simulink model "w2_warplab_trigger_proc"  (Simulink 7.7)
settings: Solver=ode45  StartTime=0.0  StopTime=1000  RelTol=1e-3
InitFcn:
  | w2_warplab_trigger_proc_init
StartFcn:
  | w2_warplab_trigger_proc_init
undefined symbols (not defined in the file or in its folder): gcbh, xlBlockLoadCallback, xlGetNormalizedPeriod
libraries: xbsIndex_r4 x819, simulink x1
(part 3 of 6)

== system w2_warplab_trigger_proc/Pulse Extender (4 cycles) ==
  IN : Inport
  Logical : xbsIndex_r4/Logical  logical_function=OR  inputs=4  en=off  latency=0  precision=Full  arith_type=Unsigned  n_bits=16  bin_pt=0  align_bp=on  dbl_ovrd=off  block_type=logical
      settings: xl_area=[1 0 0 1 0 0 0]  block_version=VER_STRING_GOES_HERE
  Register1 : xbsIndex_r4/Register  init=0  rst=off  en=off  dbl_ovrd=off  block_type=register
  Register2 : xbsIndex_r4/Register  init=0  rst=off  en=off  dbl_ovrd=off  block_type=register
  Register3 : xbsIndex_r4/Register  init=0  rst=off  en=off  dbl_ovrd=off  block_type=register
  OUT : Outport
  wires:
  Logical/1 -> OUT/1
  IN/1 -> Logical/1, Register1/1
  Register1/1 -> Logical/2, Register2/1
  Register2/1 -> Logical/3, Register3/1
  Register3/1 -> Logical/4

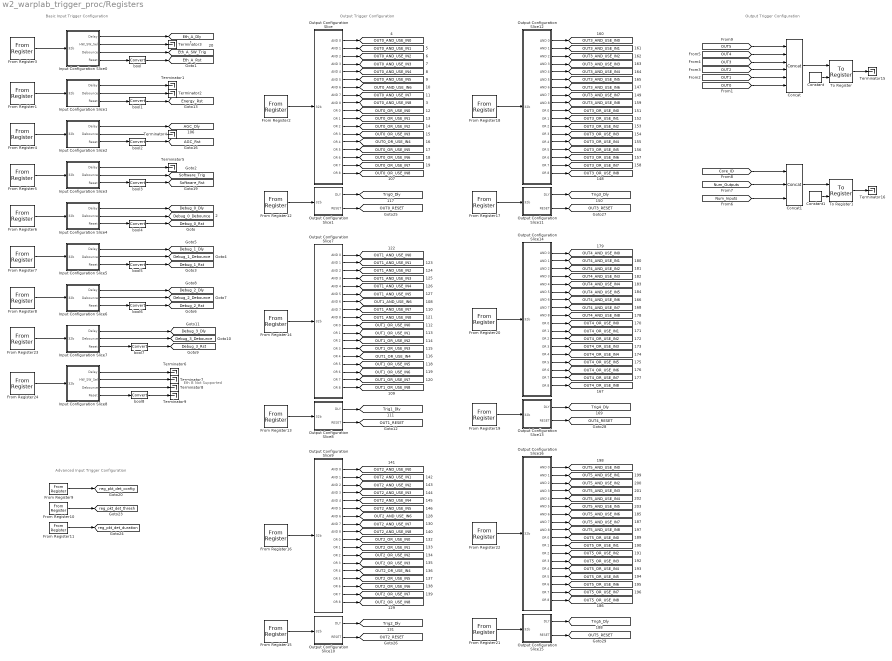
== system w2_warplab_trigger_proc/Registers ==
  note: Basic Input Trigger Configuration
  note: Advanced Input Trigger Configuration
  note: Output Trigger Configuration
  note: Output Trigger Configuration
  note: Eth B Not Supported
  Concat : xbsIndex_r4/Concat  num_inputs=6  dbl_ovrd=off  block_type=concat
  Concat1 : xbsIndex_r4/Concat  num_inputs=3  dbl_ovrd=off  block_type=concat
  Constant : xbsIndex_r4/Constant  const=1  gui_display_data_type=Boolean  arith_type=Boolean  n_bits=16  bin_pt=14  preci_type=Single  exp_width=8  frac_width=24  explicit_period=off  period=1  equ=P=C  opselect=C  inp2=PCIN>>17  opr=+  inp1=P  carry=CIN  dbl_ovrd=off  block_type=constant
  Constant1 : xbsIndex_r4/Constant  const=1  gui_display_data_type=Boolean  arith_type=Boolean  n_bits=16  bin_pt=14  preci_type=Single  exp_width=8  frac_width=24  explicit_period=off  period=1  equ=P=C  opselect=C  inp2=PCIN>>17  opr=+  inp1=P  carry=CIN  dbl_ovrd=off  block_type=constant
  From Register1 : xbsIndex_r4/From Register  shared_memory_name='TRIG_IN_CONF_1'  init=TRIG_IN_CONF_1  period=1  ownership=Locally owned and initialized  gui_display_data_type=Fixed-point  arith_type=Unsigned  n_bits=32  bin_pt=0  preci_type=Single  dbl_ovrd=off  block_type=fromreg
      settings: AttributesFormatString=<< %<shared_memory_name> >>  infoedit="Register block that reads data to a shared memory register.  Delay of one sample period."
  From Register10 : xbsIndex_r4/From Register  shared_memory_name='RSSI_PKT_DET_THRESHOLDS'  init=RSSI_PKT_DET_THRESHOLDS  period=1  ownership=Locally owned and initialized  gui_display_data_type=Fixed-point  arith_type=Unsigned  n_bits=32  bin_pt=0  preci_type=Single  dbl_ovrd=off  block_type=fromreg
      settings: AttributesFormatString=<< %<shared_memory_name> >>  infoedit="Register block that reads data to a shared memory register.  Delay of one sample period."  block_version=8.2
  From Register11 : xbsIndex_r4/From Register  shared_memory_name='RSSI_PKT_DET_DURATIONS'  init=RSSI_PKT_DET_DURATIONS  period=1  ownership=Locally owned and initialized  gui_display_data_type=Fixed-point  arith_type=Unsigned  n_bits=32  bin_pt=0  preci_type=Single  dbl_ovrd=off  block_type=fromreg
      settings: AttributesFormatString=<< %<shared_memory_name> >>  infoedit="Register block that reads data to a shared memory register.  Delay of one sample period."  block_version=8.2
  From Register12 : xbsIndex_r4/From Register  shared_memory_name='TRIG_OUT_0_CONF_1'  init=TRIG_OUT_0_CONF_1  period=1  ownership=Locally owned and initialized  gui_display_data_type=Fixed-point  arith_type=Unsigned  n_bits=32  bin_pt=0  preci_type=Single  dbl_ovrd=off  block_type=fromreg
      settings: AttributesFormatString=<< %<shared_memory_name> >>  infoedit="Register block that reads data to a shared memory register.  Delay of one sample period."
  From Register13 : xbsIndex_r4/From Register  shared_memory_name='TRIG_OUT_1_CONF_1'  init=TRIG_OUT_1_CONF_1  period=1  ownership=Locally owned and initialized  gui_display_data_type=Fixed-point  arith_type=Unsigned  n_bits=32  bin_pt=0  preci_type=Single  dbl_ovrd=off  block_type=fromreg
      settings: AttributesFormatString=<< %<shared_memory_name> >>  infoedit="Register block that reads data to a shared memory register.  Delay of one sample period."
  From Register14 : xbsIndex_r4/From Register  shared_memory_name='TRIG_OUT_1_CONF_0'  init=TRIG_OUT_1_CONF_0  period=1  ownership=Locally owned and initialized  gui_display_data_type=Fixed-point  arith_type=Unsigned  n_bits=32  bin_pt=0  preci_type=Single  dbl_ovrd=off  block_type=fromreg
      settings: AttributesFormatString=<< %<shared_memory_name> >>  infoedit="Register block that reads data to a shared memory register.  Delay of one sample period."
  From Register15 : xbsIndex_r4/From Register  shared_memory_name='TRIG_OUT_2_CONF_1'  init=TRIG_OUT_2_CONF_1  period=1  ownership=Locally owned and initialized  gui_display_data_type=Fixed-point  arith_type=Unsigned  n_bits=32  bin_pt=0  preci_type=Single  dbl_ovrd=off  block_type=fromreg
      settings: AttributesFormatString=<< %<shared_memory_name> >>  infoedit="Register block that reads data to a shared memory register.  Delay of one sample period."
  From Register16 : xbsIndex_r4/From Register  shared_memory_name='TRIG_OUT_2_CONF_0'  init=TRIG_OUT_2_CONF_0  period=1  ownership=Locally owned and initialized  gui_display_data_type=Fixed-point  arith_type=Unsigned  n_bits=32  bin_pt=0  preci_type=Single  dbl_ovrd=off  block_type=fromreg
      settings: AttributesFormatString=<< %<shared_memory_name> >>  infoedit="Register block that reads data to a shared memory register.  Delay of one sample period."
  From Register17 : xbsIndex_r4/From Register  shared_memory_name='TRIG_OUT_3_CONF_1'  init=TRIG_OUT_3_CONF_1  period=1  ownership=Locally owned and initialized  gui_display_data_type=Fixed-point  arith_type=Unsigned  n_bits=32  bin_pt=0  preci_type=Single  dbl_ovrd=off  block_type=fromreg
      settings: AttributesFormatString=<< %<shared_memory_name> >>  infoedit="Register block that reads data to a shared memory register.  Delay of one sample period."
  From Register18 : xbsIndex_r4/From Register  shared_memory_name='TRIG_OUT_3_CONF_0'  init=TRIG_OUT_3_CONF_0  period=1  ownership=Locally owned and initialized  gui_display_data_type=Fixed-point  arith_type=Unsigned  n_bits=32  bin_pt=0  preci_type=Single  dbl_ovrd=off  block_type=fromreg
      settings: AttributesFormatString=<< %<shared_memory_name> >>  infoedit="Register block that reads data to a shared memory register.  Delay of one sample period."
  From Register19 : xbsIndex_r4/From Register  shared_memory_name='TRIG_OUT_4_CONF_1'  init=TRIG_OUT_4_CONF_1  period=1  ownership=Locally owned and initialized  gui_display_data_type=Fixed-point  arith_type=Unsigned  n_bits=32  bin_pt=0  preci_type=Single  dbl_ovrd=off  block_type=fromreg
      settings: AttributesFormatString=<< %<shared_memory_name> >>  infoedit="Register block that reads data to a shared memory register.  Delay of one sample period."
  From Register2 : xbsIndex_r4/From Register  shared_memory_name='TRIG_OUT_0_CONF_0'  init=TRIG_OUT_0_CONF_0  period=1  ownership=Locally owned and initialized  gui_display_data_type=Fixed-point  arith_type=Unsigned  n_bits=32  bin_pt=0  preci_type=Single  dbl_ovrd=off  block_type=fromreg
      settings: AttributesFormatString=<< %<shared_memory_name> >>  infoedit="Register block that reads data to a shared memory register.  Delay of one sample period."
  From Register20 : xbsIndex_r4/From Register  shared_memory_name='TRIG_OUT_4_CONF_0'  init=TRIG_OUT_4_CONF_0  period=1  ownership=Locally owned and initialized  gui_display_data_type=Fixed-point  arith_type=Unsigned  n_bits=32  bin_pt=0  preci_type=Single  dbl_ovrd=off  block_type=fromreg
      settings: AttributesFormatString=<< %<shared_memory_name> >>  infoedit="Register block that reads data to a shared memory register.  Delay of one sample period."
  From Register21 : xbsIndex_r4/From Register  shared_memory_name='TRIG_OUT_5_CONF_1'  init=TRIG_OUT_5_CONF_1  period=1  ownership=Locally owned and initialized  gui_display_data_type=Fixed-point  arith_type=Unsigned  n_bits=32  bin_pt=0  preci_type=Single  dbl_ovrd=off  block_type=fromreg
      settings: AttributesFormatString=<< %<shared_memory_name> >>  infoedit="Register block that reads data to a shared memory register.  Delay of one sample period."
  From Register22 : xbsIndex_r4/From Register  shared_memory_name='TRIG_OUT_5_CONF_0'  init=TRIG_OUT_5_CONF_0  period=1  ownership=Locally owned and initialized  gui_display_data_type=Fixed-point  arith_type=Unsigned  n_bits=32  bin_pt=0  preci_type=Single  dbl_ovrd=off  block_type=fromreg
      settings: AttributesFormatString=<< %<shared_memory_name> >>  infoedit="Register block that reads data to a shared memory register.  Delay of one sample period."
  From Register23 : xbsIndex_r4/From Register  shared_memory_name='TRIG_IN_CONF_7'  init=TRIG_IN_CONF_7  period=1  ownership=Locally owned and initialized  gui_display_data_type=Fixed-point  arith_type=Unsigned  n_bits=32  bin_pt=0  preci_type=Single  dbl_ovrd=off  block_type=fromreg
      settings: AttributesFormatString=<< %<shared_memory_name> >>  infoedit="Register block that reads data to a shared memory register.  Delay of one sample period."
  From Register24 : xbsIndex_r4/From Register  shared_memory_name='TRIG_IN_CONF_8'  init=TRIG_IN_CONF_8  period=1  ownership=Locally owned and initialized  gui_display_data_type=Fixed-point  arith_type=Unsigned  n_bits=32  bin_pt=0  preci_type=Single  dbl_ovrd=off  block_type=fromreg
      settings: AttributesFormatString=<< %<shared_memory_name> >>  infoedit="Register block that reads data to a shared memory register.  Delay of one sample period."
  From Register3 : xbsIndex_r4/From Register  shared_memory_name='TRIG_IN_CONF_0'  init=TRIG_IN_CONF_0  period=1  ownership=Locally owned and initialized  gui_display_data_type=Fixed-point  arith_type=Unsigned  n_bits=32  bin_pt=0  preci_type=Single  dbl_ovrd=off  block_type=fromreg
      settings: AttributesFormatString=<< %<shared_memory_name> >>  infoedit="Register block that reads data to a shared memory register.  Delay of one sample period."
  From Register4 : xbsIndex_r4/From Register  shared_memory_name='TRIG_IN_CONF_2'  init=TRIG_IN_CONF_2  period=1  ownership=Locally owned and initialized  gui_display_data_type=Fixed-point  arith_type=Unsigned  n_bits=32  bin_pt=0  preci_type=Single  dbl_ovrd=off  block_type=fromreg
      settings: AttributesFormatString=<< %<shared_memory_name> >>  infoedit="Register block that reads data to a shared memory register.  Delay of one sample period."
  From Register5 : xbsIndex_r4/From Register  shared_memory_name='TRIG_IN_CONF_3'  init=TRIG_IN_CONF_3  period=1  ownership=Locally owned and initialized  gui_display_data_type=Fixed-point  arith_type=Unsigned  n_bits=32  bin_pt=0  preci_type=Single  dbl_ovrd=off  block_type=fromreg
      settings: AttributesFormatString=<< %<shared_memory_name> >>  infoedit="Register block that reads data to a shared memory register.  Delay of one sample period."
  From Register6 : xbsIndex_r4/From Register  shared_memory_name='TRIG_IN_CONF_4'  init=TRIG_IN_CONF_4  period=1  ownership=Locally owned and initialized  gui_display_data_type=Fixed-point  arith_type=Unsigned  n_bits=32  bin_pt=0  preci_type=Single  dbl_ovrd=off  block_type=fromreg
      settings: AttributesFormatString=<< %<shared_memory_name> >>  infoedit="Register block that reads data to a shared memory register.  Delay of one sample period."
  From Register7 : xbsIndex_r4/From Register  shared_memory_name='TRIG_IN_CONF_5'  init=TRIG_IN_CONF_5  period=1  ownership=Locally owned and initialized  gui_display_data_type=Fixed-point  arith_type=Unsigned  n_bits=32  bin_pt=0  preci_type=Single  dbl_ovrd=off  block_type=fromreg
      settings: AttributesFormatString=<< %<shared_memory_name> >>  infoedit="Register block that reads data to a shared memory register.  Delay of one sample period."
  From Register8 : xbsIndex_r4/From Register  shared_memory_name='TRIG_IN_CONF_6'  init=TRIG_IN_CONF_6  period=1  ownership=Locally owned and initialized  gui_display_data_type=Fixed-point  arith_type=Unsigned  n_bits=32  bin_pt=0  preci_type=Single  dbl_ovrd=off  block_type=fromreg
      settings: AttributesFormatString=<< %<shared_memory_name> >>  infoedit="Register block that reads data to a shared memory register.  Delay of one sample period."
  From Register9 : xbsIndex_r4/From Register  shared_memory_name='RSSI_PKT_DET_CONFIG'  init=RSSI_PKT_DET_CONFIG  period=1  ownership=Locally owned and initialized  gui_display_data_type=Fixed-point  arith_type=Unsigned  n_bits=32  bin_pt=0  preci_type=Single  dbl_ovrd=off  block_type=fromreg
      settings: AttributesFormatString=<< %<shared_memory_name> >>  infoedit="Register block that reads data to a shared memory register.  Delay of one sample period."  block_version=8.2
  Input Configuration Slice0 : Subsystem
  Input Configuration Slice1 : Subsystem
  Input Configuration Slice2 : Subsystem
  Input Configuration Slice3 : Subsystem
  Input Configuration Slice4 : Subsystem
  Input Configuration Slice5 : Subsystem
  Input Configuration Slice6 : Subsystem
  Input Configuration Slice7 : Subsystem
  Input Configuration Slice8 : Subsystem
  Output Configuration Slice : Subsystem
  Output Configuration Slice1 : Subsystem
  Output Configuration Slice10 : Subsystem
  Output Configuration Slice11 : Subsystem
  Output Configuration Slice12 : Subsystem
  Output Configuration Slice13 : Subsystem
  Output Configuration Slice14 : Subsystem
  Output Configuration Slice15 : Subsystem
  Output Configuration Slice16 : Subsystem
  Output Configuration Slice7 : Subsystem
  Output Configuration Slice8 : Subsystem
  Output Configuration Slice9 : Subsystem
  Terminator{1..9,15..16} (11 alike) : Terminator
  To Register : xbsIndex_r4/To Register  shared_memory_name='TRIG_OUT'  init=0  ownership=Locally owned and initialized  explicit_data_type=on  gui_display_data_type=Fixed-point  arith_type=Unsigned  n_bits=6  bin_pt=0  preci_type=Single  dbl_ovrd=off  block_type=toreg
      settings: AttributesFormatString=<< %<shared_memory_name> >>  infoedit="Register block that writes data to a shared memory register.  Delay of one sample period."
  To Register1 : xbsIndex_r4/To Register  shared_memory_name='CORE_INFO'  init=0  ownership=Locally owned and initialized  explicit_data_type=on  gui_display_data_type=Fixed-point  arith_type=Unsigned  n_bits=24  bin_pt=0  preci_type=Single  dbl_ovrd=off  block_type=toreg
      settings: AttributesFormatString=<< %<shared_memory_name> >>  infoedit="Register block that writes data to a shared memory register.  Delay of one sample period."
  bool{,1..8} (9 alike) : xbsIndex_r4/Convert  gui_display_data_type=Boolean  arith_type=Boolean  n_bits=16  bin_pt=14  float_type=Single  exp_bits=8  fraction_bits=24  quantization=Truncate  overflow=Wrap  en=off  latency=0  dbl_ovrd=off  pipeline=off  block_type=convert
  tag scope: AGC_Dly=global, AGC_Rst=global, Debug_0_Debounce=global, Debug_0_Dly=global, Debug_0_Rst=global, Debug_1_Debounce=global, Debug_1_Dly=global, Debug_1_Rst=global, Debug_2_Debounce=global, Debug_2_Dly=global, Debug_2_Rst=global, Debug_3_Debounce=global, Debug_3_Dly=global, Debug_3_Rst=global, Energy_Rst=global, Eth_A_Dly=global, Eth_A_Rst=global, Eth_A_SW_Trig=global, OUT0_AND_USE_IN0=global, OUT0_AND_USE_IN1=global, OUT0_AND_USE_IN2=global, OUT0_AND_USE_IN3=global, OUT0_AND_USE_IN4=global, OUT0_AND_USE_IN5=global, OUT0_AND_USE_IN6=global, OUT0_AND_USE_IN7=global, OUT0_AND_USE_IN8=global, OUT0_OR_USE_IN0=global, OUT0_OR_USE_IN1=global, OUT0_OR_USE_IN2=global, OUT0_OR_USE_IN3=global, OUT0_OR_USE_IN4=global, OUT0_OR_USE_IN5=global, OUT0_OR_USE_IN6=global, OUT0_OR_USE_IN7=global, OUT0_OR_USE_IN8=global, OUT0_RESET=global, OUT1_AND_USE_IN0=global, OUT1_AND_USE_IN1=global, OUT1_AND_USE_IN2=global, OUT1_AND_USE_IN3=global, OUT1_AND_USE_IN4=global, OUT1_AND_USE_IN5=global, OUT1_AND_USE_IN6=global, OUT1_AND_USE_IN7=global, OUT1_AND_USE_IN8=global, OUT1_OR_USE_IN0=global, OUT1_OR_USE_IN1=global, OUT1_OR_USE_IN2=global, OUT1_OR_USE_IN3=global, OUT1_OR_USE_IN4=global, OUT1_OR_USE_IN5=global, OUT1_OR_USE_IN6=global, OUT1_OR_USE_IN7=global, OUT1_OR_USE_IN8=global, OUT1_RESET=global, OUT2_AND_USE_IN0=global, OUT2_AND_USE_IN1=global, OUT2_AND_USE_IN2=global, OUT2_AND_USE_IN3=global, OUT2_AND_USE_IN4=global, OUT2_AND_USE_IN5=global, OUT2_AND_USE_IN6=global, OUT2_AND_USE_IN7=global, OUT2_AND_USE_IN8=global, OUT2_OR_USE_IN0=global, OUT2_OR_USE_IN1=global, OUT2_OR_USE_IN2=global, OUT2_OR_USE_IN3=global, OUT2_OR_USE_IN4=global, OUT2_OR_USE_IN5=global, OUT2_OR_USE_IN6=global, OUT2_OR_USE_IN7=global, OUT2_OR_USE_IN8=global, OUT2_RESET=global, OUT3_AND_USE_IN0=global, OUT3_AND_USE_IN1=global, OUT3_AND_USE_IN2=global, OUT3_AND_USE_IN3=global, OUT3_AND_USE_IN4=global, OUT3_AND_USE_IN5=global, OUT3_AND_USE_IN6=global, OUT3_AND_USE_IN7=global, OUT3_AND_USE_IN8=global, OUT3_OR_USE_IN0=global, OUT3_OR_USE_IN1=global, OUT3_OR_USE_IN2=global, OUT3_OR_USE_IN3=global, OUT3_OR_USE_IN4=global, OUT3_OR_USE_IN5=global, OUT3_OR_USE_IN6=global, OUT3_OR_USE_IN7=global, OUT3_OR_USE_IN8=global, OUT3_RESET=global, OUT4_AND_USE_IN0=global, OUT4_AND_USE_IN1=global, OUT4_AND_USE_IN2=global, OUT4_AND_USE_IN3=global, OUT4_AND_USE_IN4=global, OUT4_AND_USE_IN5=global, OUT4_AND_USE_IN6=global, OUT4_AND_USE_IN7=global, OUT4_AND_USE_IN8=global, OUT4_OR_USE_IN0=global, OUT4_OR_USE_IN1=global, OUT4_OR_USE_IN2=global, OUT4_OR_USE_IN3=global, OUT4_OR_USE_IN4=global, OUT4_OR_USE_IN5=global, OUT4_OR_USE_IN6=global, OUT4_OR_USE_IN7=global, OUT4_OR_USE_IN8=global, OUT4_RESET=global, OUT5_AND_USE_IN0=global, OUT5_AND_USE_IN1=global, OUT5_AND_USE_IN2=global, OUT5_AND_USE_IN3=global, OUT5_AND_USE_IN4=global, OUT5_AND_USE_IN5=global, OUT5_AND_USE_IN6=global, OUT5_AND_USE_IN7=global, OUT5_AND_USE_IN8=global, OUT5_OR_USE_IN0=global, OUT5_OR_USE_IN1=global, OUT5_OR_USE_IN2=global, OUT5_OR_USE_IN3=global, OUT5_OR_USE_IN4=global, OUT5_OR_USE_IN5=global, OUT5_OR_USE_IN6=global, OUT5_OR_USE_IN7=global, OUT5_OR_USE_IN8=global, OUT5_RESET=global, Software_Rst=global, Software_Trig=global, Trig0_Dly=global, Trig1_Dly=global, Trig2_Dly=global, Trig3_Dly=global, Trig4_Dly=global, Trig5_Dly=global, reg_pkt_det_config=global, reg_pkt_det_duration=global, reg_pkt_det_thresh=global
  wires:
  From Register9/1 -> [reg_pkt_det_config]
  From Register10/1 -> [reg_pkt_det_thresh]
  From Register11/1 -> [reg_pkt_det_duration]
  From Register2/1 -> Output Configuration Slice/1(32b)
  Output Configuration Slice/1(AND 0) -> [OUT0_AND_USE_IN0]
  Output Configuration Slice/2(AND 1) -> [OUT0_AND_USE_IN1]
  Output Configuration Slice/3(AND 2) -> [OUT0_AND_USE_IN2]
  Output Configuration Slice/4(AND 3) -> [OUT0_AND_USE_IN3]
  Output Configuration Slice/5(AND 4) -> [OUT0_AND_USE_IN4]
  Output Configuration Slice/6(AND 5) -> [OUT0_AND_USE_IN5]
  Output Configuration Slice/7(AND 6) -> [OUT0_AND_USE_IN6]
  Output Configuration Slice/8(AND 7) -> [OUT0_AND_USE_IN7]
  Output Configuration Slice/10(OR 0) -> [OUT0_OR_USE_IN0]
  Output Configuration Slice/11(OR 1) -> [OUT0_OR_USE_IN1]
  Output Configuration Slice/12(OR 2) -> [OUT0_OR_USE_IN2]
  Output Configuration Slice/13(OR 3) -> [OUT0_OR_USE_IN3]
  Output Configuration Slice/14(OR 4) -> [OUT0_OR_USE_IN4]
  Output Configuration Slice/15(OR 5) -> [OUT0_OR_USE_IN5]
  Output Configuration Slice/16(OR 6) -> [OUT0_OR_USE_IN6]
  Output Configuration Slice/17(OR 7) -> [OUT0_OR_USE_IN7]
  [OUT4] -> Concat/2
  [OUT3] -> Concat/3
  [OUT2] -> Concat/4
  [OUT1] -> Concat/5
  [OUT0] -> Concat/6
  Concat/1 -> To Register/1
  Constant/1 -> To Register/2
  Concat1/1 -> To Register1/1
  Constant1/1 -> To Register1/2
  [Core_ID] -> Concat1/1
  [Num_Outputs] -> Concat1/2
  [Num_Inputs] -> Concat1/3
  Output Configuration Slice/9(AND 8) -> [OUT0_AND_USE_IN8]
  Output Configuration Slice/18(OR 8) -> [OUT0_OR_USE_IN8]
  From Register14/1 -> Output Configuration Slice7/1(32b)
  Output Configuration Slice7/1(AND 0) -> [OUT1_AND_USE_IN0]
  Output Configuration Slice7/2(AND 1) -> [OUT1_AND_USE_IN1]
  Output Configuration Slice7/3(AND 2) -> [OUT1_AND_USE_IN2]
  Output Configuration Slice7/4(AND 3) -> [OUT1_AND_USE_IN3]
  Output Configuration Slice7/5(AND 4) -> [OUT1_AND_USE_IN4]
  Output Configuration Slice7/6(AND 5) -> [OUT1_AND_USE_IN5]
  Output Configuration Slice7/7(AND 6) -> [OUT1_AND_USE_IN6]
  Output Configuration Slice7/8(AND 7) -> [OUT1_AND_USE_IN7]
  Output Configuration Slice7/10(OR 0) -> [OUT1_OR_USE_IN0]
  Output Configuration Slice7/11(OR 1) -> [OUT1_OR_USE_IN1]
  Output Configuration Slice7/12(OR 2) -> [OUT1_OR_USE_IN2]
  Output Configuration Slice7/13(OR 3) -> [OUT1_OR_USE_IN3]
  Output Configuration Slice7/14(OR 4) -> [OUT1_OR_USE_IN4]
  Output Configuration Slice7/15(OR 5) -> [OUT1_OR_USE_IN5]
  Output Configuration Slice7/16(OR 6) -> [OUT1_OR_USE_IN6]
  Output Configuration Slice7/17(OR 7) -> [OUT1_OR_USE_IN7]
  From Register13/1 -> Output Configuration Slice8/1(32b)
  Output Configuration Slice8/2(RESET) -> [OUT1_RESET]
  Output Configuration Slice8/1(DLY) -> [Trig1_Dly]
  Output Configuration Slice7/9(AND 8) -> [OUT1_AND_USE_IN8]
  Output Configuration Slice7/18(OR 8) -> [OUT1_OR_USE_IN8]
  From Register16/1 -> Output Configuration Slice9/1(32b)
  Output Configuration Slice9/1(AND 0) -> [OUT2_AND_USE_IN0]
  Output Configuration Slice9/2(AND 1) -> [OUT2_AND_USE_IN1]
  Output Configuration Slice9/3(AND 2) -> [OUT2_AND_USE_IN2]
  Output Configuration Slice9/4(AND 3) -> [OUT2_AND_USE_IN3]
  Output Configuration Slice9/5(AND 4) -> [OUT2_AND_USE_IN4]
  Output Configuration Slice9/6(AND 5) -> [OUT2_AND_USE_IN5]
  Output Configuration Slice9/7(AND 6) -> [OUT2_AND_USE_IN6]
  Output Configuration Slice9/8(AND 7) -> [OUT2_AND_USE_IN7]
  Output Configuration Slice9/10(OR 0) -> [OUT2_OR_USE_IN0]
  Output Configuration Slice9/11(OR 1) -> [OUT2_OR_USE_IN1]
  Output Configuration Slice9/12(OR 2) -> [OUT2_OR_USE_IN2]
  Output Configuration Slice9/13(OR 3) -> [OUT2_OR_USE_IN3]
  Output Configuration Slice9/14(OR 4) -> [OUT2_OR_USE_IN4]
  Output Configuration Slice9/15(OR 5) -> [OUT2_OR_USE_IN5]
  Output Configuration Slice9/16(OR 6) -> [OUT2_OR_USE_IN6]
  Output Configuration Slice9/17(OR 7) -> [OUT2_OR_USE_IN7]
  From Register15/1 -> Output Configuration Slice10/1(32b)
  Output Configuration Slice10/2(RESET) -> [OUT2_RESET]
  Output Configuration Slice10/1(DLY) -> [Trig2_Dly]
  Output Configuration Slice9/9(AND 8) -> [OUT2_AND_USE_IN8]
  Output Configuration Slice9/18(OR 8) -> [OUT2_OR_USE_IN8]
  From Register18/1 -> Output Configuration Slice12/1(32b)
  Output Configuration Slice12/1(AND 0) -> [OUT3_AND_USE_IN0]
  Output Configuration Slice12/2(AND 1) -> [OUT3_AND_USE_IN1]
  Output Configuration Slice12/3(AND 2) -> [OUT3_AND_USE_IN2]
  Output Configuration Slice12/4(AND 3) -> [OUT3_AND_USE_IN3]
  Output Configuration Slice12/5(AND 4) -> [OUT3_AND_USE_IN4]
  Output Configuration Slice12/6(AND 5) -> [OUT3_AND_USE_IN5]
  Output Configuration Slice12/7(AND 6) -> [OUT3_AND_USE_IN6]
  Output Configuration Slice12/8(AND 7) -> [OUT3_AND_USE_IN7]
  Output Configuration Slice12/10(OR 0) -> [OUT3_OR_USE_IN0]
  Output Configuration Slice12/11(OR 1) -> [OUT3_OR_USE_IN1]
  Output Configuration Slice12/12(OR 2) -> [OUT3_OR_USE_IN2]
  Output Configuration Slice12/13(OR 3) -> [OUT3_OR_USE_IN3]
  Output Configuration Slice12/14(OR 4) -> [OUT3_OR_USE_IN4]
  Output Configuration Slice12/15(OR 5) -> [OUT3_OR_USE_IN5]
  Output Configuration Slice12/16(OR 6) -> [OUT3_OR_USE_IN6]
  Output Configuration Slice12/17(OR 7) -> [OUT3_OR_USE_IN7]
  From Register17/1 -> Output Configuration Slice11/1(32b)
  Output Configuration Slice11/2(RESET) -> [OUT3_RESET]
  Output Configuration Slice11/1(DLY) -> [Trig3_Dly]
  Output Configuration Slice12/9(AND 8) -> [OUT3_AND_USE_IN8]
  Output Configuration Slice12/18(OR 8) -> [OUT3_OR_USE_IN8]
  From Register20/1 -> Output Configuration Slice14/1(32b)
  Output Configuration Slice14/1(AND 0) -> [OUT4_AND_USE_IN0]
  Output Configuration Slice14/2(AND 1) -> [OUT4_AND_USE_IN1]
  Output Configuration Slice14/3(AND 2) -> [OUT4_AND_USE_IN2]
  Output Configuration Slice14/4(AND 3) -> [OUT4_AND_USE_IN3]
  Output Configuration Slice14/5(AND 4) -> [OUT4_AND_USE_IN4]
  Output Configuration Slice14/6(AND 5) -> [OUT4_AND_USE_IN5]
  Output Configuration Slice14/7(AND 6) -> [OUT4_AND_USE_IN6]
  Output Configuration Slice14/8(AND 7) -> [OUT4_AND_USE_IN7]
  Output Configuration Slice14/10(OR 0) -> [OUT4_OR_USE_IN0]
  Output Configuration Slice14/11(OR 1) -> [OUT4_OR_USE_IN1]
  Output Configuration Slice14/12(OR 2) -> [OUT4_OR_USE_IN2]
  Output Configuration Slice14/13(OR 3) -> [OUT4_OR_USE_IN3]
  Output Configuration Slice14/14(OR 4) -> [OUT4_OR_USE_IN4]
  Output Configuration Slice14/15(OR 5) -> [OUT4_OR_USE_IN5]
  Output Configuration Slice14/16(OR 6) -> [OUT4_OR_USE_IN6]
  Output Configuration Slice14/17(OR 7) -> [OUT4_OR_USE_IN7]
  From Register19/1 -> Output Configuration Slice13/1(32b)
  Output Configuration Slice13/2(RESET) -> [OUT4_RESET]
  Output Configuration Slice13/1(DLY) -> [Trig4_Dly]
  Output Configuration Slice14/9(AND 8) -> [OUT4_AND_USE_IN8]
  Output Configuration Slice14/18(OR 8) -> [OUT4_OR_USE_IN8]
  From Register22/1 -> Output Configuration Slice16/1(32b)
  Output Configuration Slice16/1(AND 0) -> [OUT5_AND_USE_IN0]
  Output Configuration Slice16/2(AND 1) -> [OUT5_AND_USE_IN1]
  Output Configuration Slice16/3(AND 2) -> [OUT5_AND_USE_IN2]
  Output Configuration Slice16/4(AND 3) -> [OUT5_AND_USE_IN3]
  Output Configuration Slice16/5(AND 4) -> [OUT5_AND_USE_IN4]
  Output Configuration Slice16/6(AND 5) -> [OUT5_AND_USE_IN5]
  Output Configuration Slice16/7(AND 6) -> [OUT5_AND_USE_IN6]
  Output Configuration Slice16/8(AND 7) -> [OUT5_AND_USE_IN7]
  Output Configuration Slice16/10(OR 0) -> [OUT5_OR_USE_IN0]
  Output Configuration Slice16/11(OR 1) -> [OUT5_OR_USE_IN1]
  Output Configuration Slice16/12(OR 2) -> [OUT5_OR_USE_IN2]
  Output Configuration Slice16/13(OR 3) -> [OUT5_OR_USE_IN3]
  Output Configuration Slice16/14(OR 4) -> [OUT5_OR_USE_IN4]
  Output Configuration Slice16/15(OR 5) -> [OUT5_OR_USE_IN5]
  Output Configuration Slice16/16(OR 6) -> [OUT5_OR_USE_IN6]
  Output Configuration Slice16/17(OR 7) -> [OUT5_OR_USE_IN7]
  From Register21/1 -> Output Configuration Slice15/1(32b)
  Output Configuration Slice15/2(RESET) -> [OUT5_RESET]
  Output Configuration Slice15/1(DLY) -> [Trig5_Dly]
  Output Configuration Slice16/9(AND 8) -> [OUT5_AND_USE_IN8]
  Output Configuration Slice16/18(OR 8) -> [OUT5_OR_USE_IN8]
  Output Configuration Slice1/1(DLY) -> [Trig0_Dly]
  Output Configuration Slice1/2(RESET) -> [OUT0_RESET]
  From Register12/1 -> Output Configuration Slice1/1(32b)
  To Register/1 -> Terminator15/1
  To Register1/1 -> Terminator16/1
  [OUT5] -> Concat/1
  bool/1 -> [Eth_A_Rst]
  bool1/1 -> [Energy_Rst]
  bool2/1 -> [AGC_Rst]
  bool3/1 -> [Software_Rst]
  bool4/1 -> [Debug_0_Rst]
  bool5/1 -> [Debug_1_Rst]
  bool6/1 -> [Debug_2_Rst]
  bool7/1 -> [Debug_3_Rst]
  bool8/1 -> Terminator9/1
  From Register3/1 -> Input Configuration Slice0/1(32b)
  From Register1/1 -> Input Configuration Slice1/1(32b)
  From Register4/1 -> Input Configuration Slice2/1(32b)
  From Register5/1 -> Input Configuration Slice3/1(32b)
  From Register6/1 -> Input Configuration Slice4/1(32b)
  Input Configuration Slice0/1(Delay) -> [Eth_A_Dly]
  Input Configuration Slice0/3(Debounce) -> [Eth_A_SW_Trig]
  Input Configuration Slice0/4(Reset) -> bool/1
  From Register7/1 -> Input Configuration Slice5/1(32b)
  From Register8/1 -> Input Configuration Slice6/1(32b)
  From Register23/1 -> Input Configuration Slice7/1(32b)
  From Register24/1 -> Input Configuration Slice8/1(32b)
  Input Configuration Slice1/1(Delay) -> Terminator1/1
  Input Configuration Slice1/2(Debounce) -> Terminator2/1
  Input Configuration Slice1/3(Reset) -> bool1/1
  Input Configuration Slice2/1(Delay) -> [AGC_Dly]
  Input Configuration Slice2/2(Debounce) -> Terminator4/1
  Input Configuration Slice2/3(Reset) -> bool2/1
  Input Configuration Slice3/1(Delay) -> Terminator5/1
  Input Configuration Slice3/2(Debounce) -> [Software_Trig]
  Input Configuration Slice3/3(Reset) -> bool3/1
  Input Configuration Slice4/1(Delay) -> [Debug_0_Dly]
  Input Configuration Slice4/2(Debounce) -> [Debug_0_Debounce]
  Input Configuration Slice4/3(Reset) -> bool4/1
  Input Configuration Slice5/1(Delay) -> [Debug_1_Dly]
  Input Configuration Slice5/2(Debounce) -> [Debug_1_Debounce]
  Input Configuration Slice5/3(Reset) -> bool5/1
  Input Configuration Slice6/1(Delay) -> [Debug_2_Dly]
  Input Configuration Slice6/2(Debounce) -> [Debug_2_Debounce]
  Input Configuration Slice6/3(Reset) -> bool6/1
  Input Configuration Slice7/1(Delay) -> [Debug_3_Dly]
  Input Configuration Slice7/2(Debounce) -> [Debug_3_Debounce]
  Input Configuration Slice7/3(Reset) -> bool7/1
  Input Configuration Slice0/2(HW_SW_Sel) -> Terminator3/1
  Input Configuration Slice8/1(Delay) -> Terminator6/1
  Input Configuration Slice8/2(HW_SW_Sel) -> Terminator7/1
  Input Configuration Slice8/3(Debounce) -> Terminator8/1
  Input Configuration Slice8/4(Reset) -> bool8/1

== system w2_warplab_trigger_proc/RisingEdge ==
  IN : Inport
  Delay : xbsIndex_r4/Delay  rst=off  infoeditControl=Selection of Reset will increase slice count due to use of real FFs and instead of SRLs  en=off  latency=1  dbl_ovrd=off  reg_retiming=off  block_type=delay
      settings: infoedit=Hardware notes: A delay line is a chain, each link of which is an SRL16 followed by a flip-flop. If register retiming is enabled, the delay line is a chain of flip-flops.  xl_area=[1 1 0 0 0 0 0]  block_version=VER_STRING_GOES_HERE
  Inverter : xbsIndex_r4/Inverter  en=off  latency=0  dbl_ovrd=off  block_type=inv
      settings: xl_area=[0 0 0 0 0 0 0]  block_version=VER_STRING_GOES_HERE
  Logical : xbsIndex_r4/Logical  logical_function=AND  inputs=2  en=off  latency=0  precision=Full  arith_type=Unsigned  n_bits=16  bin_pt=0  align_bp=on  dbl_ovrd=off  block_type=logical
      settings: xl_area=[1 0 0 1 0 0 0]  block_version=VER_STRING_GOES_HERE
  Edge : Outport
  wires:
  Logical/1 -> Edge/1
  Delay/1 -> Logical/2
  Inverter/1 -> Delay/1
  IN/1 -> Logical/1, Inverter/1

== system w2_warplab_trigger_proc/S-R Latch ==
  S : Inport
  R : Inport  Port=2
  Constant1 : xbsIndex_r4/Constant  const=1  gui_display_data_type=Boolean  arith_type=Boolean  n_bits=1  bin_pt=0  preci_type=Single  exp_width=8  frac_width=24  explicit_period=off  period=1  equ=P=C  opselect=C  inp2=PCIN>>17  opr=+  inp1=P  carry=CIN  dbl_ovrd=off  block_type=constant
      settings: block_version=VER_STRING_GOES_HERE
  Convert1 : xbsIndex_r4/Convert  gui_display_data_type=Boolean  arith_type=Boolean  n_bits=1  bin_pt=0  float_type=Single  exp_bits=8  fraction_bits=24  quantization=Truncate  overflow=Wrap  en=off  latency=0  dbl_ovrd=off  pipeline=off  block_type=convert
  Convert2 : xbsIndex_r4/Convert  gui_display_data_type=Boolean  arith_type=Boolean  n_bits=1  bin_pt=0  float_type=Single  exp_bits=8  fraction_bits=24  quantization=Truncate  overflow=Wrap  en=off  latency=0  dbl_ovrd=off  pipeline=off  block_type=convert
  Register2 : xbsIndex_r4/Register  init=0  rst=on  en=on  dbl_ovrd=off  block_type=register
      settings: xl_area=[1 1 0 0 0 0 0]  block_version=VER_STRING_GOES_HERE
  Q : Outport
  wires:
  S/1 -> Convert2/1
  Register2/1 -> Q/1
  R/1 -> Convert1/1
  Constant1/1 -> Register2/1
  Convert1/1 -> Register2/2
  Convert2/1 -> Register2/3

== system w2_warplab_trigger_proc/S-R Latch1 ==
  S : Inport
  R : Inport  Port=2
  Constant1 : xbsIndex_r4/Constant  const=1  gui_display_data_type=Boolean  arith_type=Boolean  n_bits=1  bin_pt=0  preci_type=Single  exp_width=8  frac_width=24  explicit_period=off  period=1  equ=P=C  opselect=C  inp2=PCIN>>17  opr=+  inp1=P  carry=CIN  dbl_ovrd=off  block_type=constant
      settings: block_version=VER_STRING_GOES_HERE
  Convert1 : xbsIndex_r4/Convert  gui_display_data_type=Boolean  arith_type=Boolean  n_bits=1  bin_pt=0  float_type=Single  exp_bits=8  fraction_bits=24  quantization=Truncate  overflow=Wrap  en=off  latency=0  dbl_ovrd=off  pipeline=off  block_type=convert
  Convert2 : xbsIndex_r4/Convert  gui_display_data_type=Boolean  arith_type=Boolean  n_bits=1  bin_pt=0  float_type=Single  exp_bits=8  fraction_bits=24  quantization=Truncate  overflow=Wrap  en=off  latency=0  dbl_ovrd=off  pipeline=off  block_type=convert
  Register2 : xbsIndex_r4/Register  init=0  rst=on  en=on  dbl_ovrd=off  block_type=register
      settings: xl_area=[1 1 0 0 0 0 0]  block_version=VER_STRING_GOES_HERE
  Q : Outport
  wires:
  S/1 -> Convert2/1
  Register2/1 -> Q/1
  R/1 -> Convert1/1
  Constant1/1 -> Register2/1
  Convert1/1 -> Register2/2
  Convert2/1 -> Register2/3

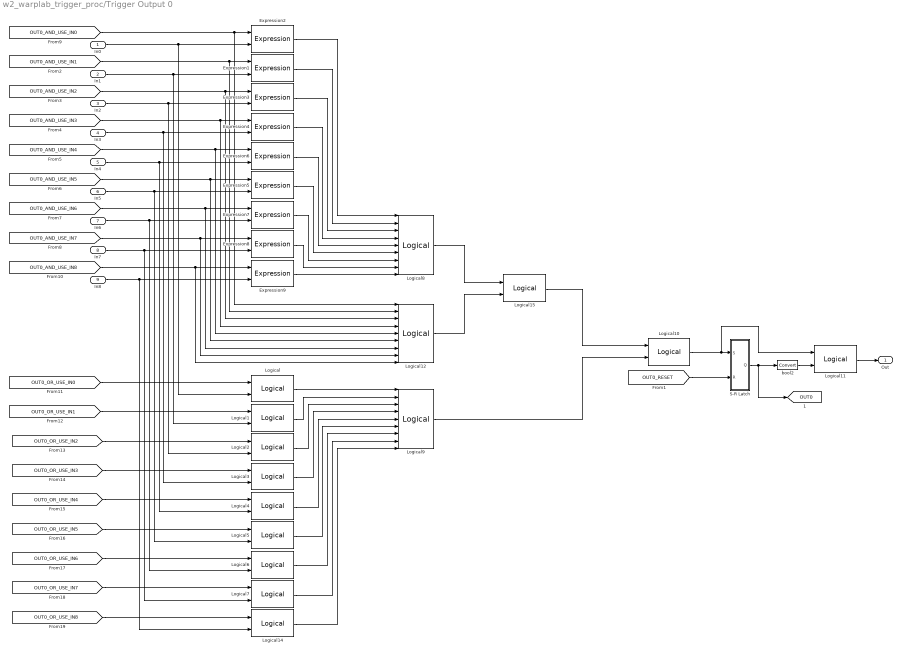
== system w2_warplab_trigger_proc/Trigger Output 0 ==
  In0 : Inport
  In1 : Inport  Port=2
  In2 : Inport  Port=3
  In3 : Inport  Port=4
  In4 : Inport  Port=5
  In5 : Inport  Port=6
  In6 : Inport  Port=7
  In7 : Inport  Port=8
  In8 : Inport  Port=9
  Expression{1..9} (9 alike) : xbsIndex_r4/Expression  expression=~a | (a & b)  align_bp=on  en=off  latency=0  precision=Full  arith_type=Unsigned  n_bits=16  bin_pt=0  dbl_ovrd=off  block_type=expr
  Logical{,1..7,14..15} (10 alike) : xbsIndex_r4/Logical  logical_function=AND  inputs=2  en=off  latency=0  precision=Full  arith_type=Unsigned  n_bits=16  bin_pt=0  align_bp=on  dbl_ovrd=off  block_type=logical
  Logical10 : xbsIndex_r4/Logical  logical_function=OR  inputs=2  en=off  latency=0  precision=Full  arith_type=Unsigned  n_bits=16  bin_pt=0  align_bp=on  dbl_ovrd=off  block_type=logical
  Logical11 : xbsIndex_r4/Logical  logical_function=OR  inputs=2  en=off  latency=0  precision=Full  arith_type=Unsigned  n_bits=16  bin_pt=0  align_bp=on  dbl_ovrd=off  block_type=logical
  Logical12 : xbsIndex_r4/Logical  logical_function=OR  inputs=9  en=off  latency=0  precision=Full  arith_type=Unsigned  n_bits=16  bin_pt=0  align_bp=on  dbl_ovrd=off  block_type=logical
  Logical8 : xbsIndex_r4/Logical  logical_function=AND  inputs=9  en=off  latency=0  precision=Full  arith_type=Unsigned  n_bits=16  bin_pt=0  align_bp=on  dbl_ovrd=off  block_type=logical
  Logical9 : xbsIndex_r4/Logical  logical_function=OR  inputs=9  en=off  latency=0  precision=Full  arith_type=Unsigned  n_bits=16  bin_pt=0  align_bp=on  dbl_ovrd=off  block_type=logical
  S-R Latch : Subsystem
  bool2 : xbsIndex_r4/Convert  gui_display_data_type=Boolean  arith_type=Boolean  n_bits=16  bin_pt=14  float_type=Single  exp_bits=8  fraction_bits=24  quantization=Truncate  overflow=Wrap  en=off  latency=0  dbl_ovrd=off  pipeline=off  block_type=convert
  Out : Outport
  tag scope: OUT0=global
  wires:
  [OUT0_AND_USE_IN0] -> Expression2/1, Logical12/1
  [OUT0_AND_USE_IN1] -> Expression1/1, Logical12/2
  [OUT0_AND_USE_IN2] -> Expression3/1, Logical12/3
  [OUT0_AND_USE_IN3] -> Expression4/1, Logical12/4
  [OUT0_AND_USE_IN4] -> Expression6/1, Logical12/5
  [OUT0_AND_USE_IN5] -> Expression5/1, Logical12/6
  [OUT0_AND_USE_IN6] -> Expression7/1, Logical12/7
  [OUT0_AND_USE_IN7] -> Expression8/1, Logical12/8
  In0/1 -> Logical/2, Expression2/2
  In1/1 -> Expression1/2, Logical1/2
  In2/1 -> Expression3/2, Logical2/2
  In3/1 -> Expression4/2, Logical3/2
  In4/1 -> Expression6/2, Logical4/2
  In5/1 -> Expression5/2, Logical5/2
  In6/1 -> Expression7/2, Logical6/2
  In7/1 -> Expression8/2, Logical7/2
  [OUT0_OR_USE_IN0] -> Logical/1
  [OUT0_OR_USE_IN1] -> Logical1/1
  Expression2/1 -> Logical8/1
  Expression1/1 -> Logical8/2
  Expression3/1 -> Logical8/3
  Expression4/1 -> Logical8/4
  Expression6/1 -> Logical8/5
  Expression5/1 -> Logical8/6
  Expression7/1 -> Logical8/7
  Expression8/1 -> Logical8/8
  Logical1/1 -> Logical9/2
  Logical2/1 -> Logical9/3
  Logical3/1 -> Logical9/4
  Logical4/1 -> Logical9/5
  Logical5/1 -> Logical9/6
  Logical6/1 -> Logical9/7
  Logical7/1 -> Logical9/8
  Logical9/1 -> Logical10/2
  Logical10/1 -> S-R Latch/1(S), Logical11/1
  [OUT0_RESET] -> S-R Latch/2(R)
  S-R Latch/1(Q) -> [OUT0], bool2/1
  Logical11/1 -> Out/1
  bool2/1 -> Logical11/2
  Logical12/1 -> Logical15/2
  Logical15/1 -> Logical10/1
  [OUT0_AND_USE_IN8] -> Expression9/1, Logical12/9
  In8/1 -> Expression9/2, Logical14/2
  Logical8/1 -> Logical15/1
  [OUT0_OR_USE_IN2] -> Logical2/1
  [OUT0_OR_USE_IN3] -> Logical3/1
  [OUT0_OR_USE_IN4] -> Logical4/1
  [OUT0_OR_USE_IN5] -> Logical5/1
  [OUT0_OR_USE_IN6] -> Logical6/1
  [OUT0_OR_USE_IN7] -> Logical7/1
  [OUT0_OR_USE_IN8] -> Logical14/1
  Logical14/1 -> Logical9/9
  Expression9/1 -> Logical8/9
  Logical/1 -> Logical9/1

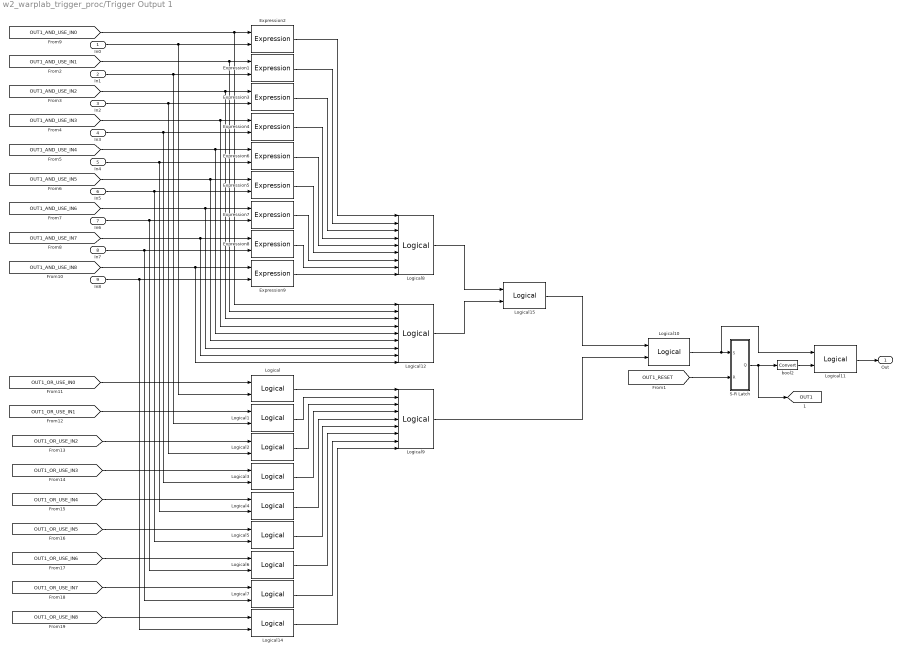
== system w2_warplab_trigger_proc/Trigger Output 1 ==
  In0 : Inport
  In1 : Inport  Port=2
  In2 : Inport  Port=3
  In3 : Inport  Port=4
  In4 : Inport  Port=5
  In5 : Inport  Port=6
  In6 : Inport  Port=7
  In7 : Inport  Port=8
  In8 : Inport  Port=9
  Expression{1..9} (9 alike) : xbsIndex_r4/Expression  expression=~a | (a & b)  align_bp=on  en=off  latency=0  precision=Full  arith_type=Unsigned  n_bits=16  bin_pt=0  dbl_ovrd=off  block_type=expr
  Logical{,1..7,14..15} (10 alike) : xbsIndex_r4/Logical  logical_function=AND  inputs=2  en=off  latency=0  precision=Full  arith_type=Unsigned  n_bits=16  bin_pt=0  align_bp=on  dbl_ovrd=off  block_type=logical
  Logical10 : xbsIndex_r4/Logical  logical_function=OR  inputs=2  en=off  latency=0  precision=Full  arith_type=Unsigned  n_bits=16  bin_pt=0  align_bp=on  dbl_ovrd=off  block_type=logical
  Logical11 : xbsIndex_r4/Logical  logical_function=OR  inputs=2  en=off  latency=0  precision=Full  arith_type=Unsigned  n_bits=16  bin_pt=0  align_bp=on  dbl_ovrd=off  block_type=logical
  Logical12 : xbsIndex_r4/Logical  logical_function=OR  inputs=9  en=off  latency=0  precision=Full  arith_type=Unsigned  n_bits=16  bin_pt=0  align_bp=on  dbl_ovrd=off  block_type=logical
  Logical8 : xbsIndex_r4/Logical  logical_function=AND  inputs=9  en=off  latency=0  precision=Full  arith_type=Unsigned  n_bits=16  bin_pt=0  align_bp=on  dbl_ovrd=off  block_type=logical
  Logical9 : xbsIndex_r4/Logical  logical_function=OR  inputs=9  en=off  latency=0  precision=Full  arith_type=Unsigned  n_bits=16  bin_pt=0  align_bp=on  dbl_ovrd=off  block_type=logical
  S-R Latch : Subsystem
  bool2 : xbsIndex_r4/Convert  gui_display_data_type=Boolean  arith_type=Boolean  n_bits=16  bin_pt=14  float_type=Single  exp_bits=8  fraction_bits=24  quantization=Truncate  overflow=Wrap  en=off  latency=0  dbl_ovrd=off  pipeline=off  block_type=convert
  Out : Outport
  tag scope: OUT1=global
  wires:
  [OUT1_AND_USE_IN0] -> Expression2/1, Logical12/1
  [OUT1_AND_USE_IN1] -> Expression1/1, Logical12/2
  [OUT1_AND_USE_IN2] -> Expression3/1, Logical12/3
  [OUT1_AND_USE_IN3] -> Expression4/1, Logical12/4
  [OUT1_AND_USE_IN4] -> Expression6/1, Logical12/5
  [OUT1_AND_USE_IN5] -> Expression5/1, Logical12/6
  [OUT1_AND_USE_IN6] -> Expression7/1, Logical12/7
  [OUT1_AND_USE_IN7] -> Expression8/1, Logical12/8
  In0/1 -> Logical/2, Expression2/2
  In1/1 -> Expression1/2, Logical1/2
  In2/1 -> Expression3/2, Logical2/2
  In3/1 -> Expression4/2, Logical3/2
  In4/1 -> Expression6/2, Logical4/2
  In5/1 -> Expression5/2, Logical5/2
  In6/1 -> Expression7/2, Logical6/2
  In7/1 -> Expression8/2, Logical7/2
  [OUT1_OR_USE_IN0] -> Logical/1
  [OUT1_OR_USE_IN1] -> Logical1/1
  Expression2/1 -> Logical8/1
  Expression1/1 -> Logical8/2
  Expression3/1 -> Logical8/3
  Expression4/1 -> Logical8/4
  Expression6/1 -> Logical8/5
  Expression5/1 -> Logical8/6
  Expression7/1 -> Logical8/7
  Expression8/1 -> Logical8/8
  Logical/1 -> Logical9/1
  Logical1/1 -> Logical9/2
  Logical2/1 -> Logical9/3
  Logical3/1 -> Logical9/4
  Logical4/1 -> Logical9/5
  Logical5/1 -> Logical9/6
  Logical6/1 -> Logical9/7
  Logical7/1 -> Logical9/8
  Logical9/1 -> Logical10/2
  Logical10/1 -> S-R Latch/1(S), Logical11/1
  [OUT1_RESET] -> S-R Latch/2(R)
  S-R Latch/1(Q) -> [OUT1], bool2/1
  Logical11/1 -> Out/1
  bool2/1 -> Logical11/2
  Logical12/1 -> Logical15/2
  Logical15/1 -> Logical10/1
  [OUT1_AND_USE_IN8] -> Expression9/1, Logical12/9
  In8/1 -> Expression9/2, Logical14/2
  Logical8/1 -> Logical15/1
  Expression9/1 -> Logical8/9
  [OUT1_OR_USE_IN2] -> Logical2/1
  [OUT1_OR_USE_IN3] -> Logical3/1
  [OUT1_OR_USE_IN4] -> Logical4/1
  [OUT1_OR_USE_IN5] -> Logical5/1
  [OUT1_OR_USE_IN6] -> Logical6/1
  [OUT1_OR_USE_IN7] -> Logical7/1
  [OUT1_OR_USE_IN8] -> Logical14/1
  Logical14/1 -> Logical9/9

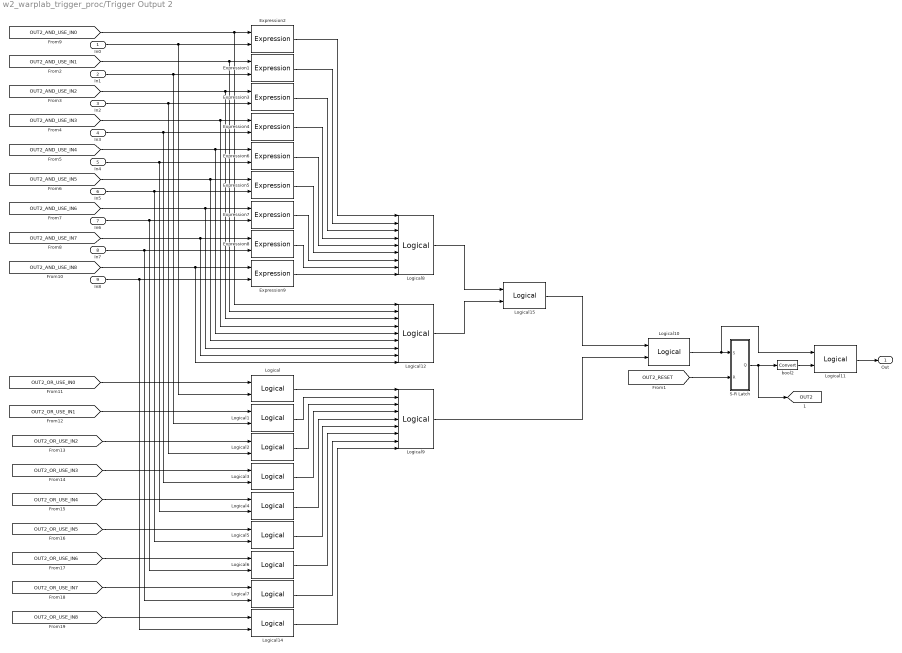
== system w2_warplab_trigger_proc/Trigger Output 2 ==
  In0 : Inport
  In1 : Inport  Port=2
  In2 : Inport  Port=3
  In3 : Inport  Port=4
  In4 : Inport  Port=5
  In5 : Inport  Port=6
  In6 : Inport  Port=7
  In7 : Inport  Port=8
  In8 : Inport  Port=9
  Expression{1..9} (9 alike) : xbsIndex_r4/Expression  expression=~a | (a & b)  align_bp=on  en=off  latency=0  precision=Full  arith_type=Unsigned  n_bits=16  bin_pt=0  dbl_ovrd=off  block_type=expr
  Logical{,1..7,14..15} (10 alike) : xbsIndex_r4/Logical  logical_function=AND  inputs=2  en=off  latency=0  precision=Full  arith_type=Unsigned  n_bits=16  bin_pt=0  align_bp=on  dbl_ovrd=off  block_type=logical
  Logical10 : xbsIndex_r4/Logical  logical_function=OR  inputs=2  en=off  latency=0  precision=Full  arith_type=Unsigned  n_bits=16  bin_pt=0  align_bp=on  dbl_ovrd=off  block_type=logical
  Logical11 : xbsIndex_r4/Logical  logical_function=OR  inputs=2  en=off  latency=0  precision=Full  arith_type=Unsigned  n_bits=16  bin_pt=0  align_bp=on  dbl_ovrd=off  block_type=logical
  Logical12 : xbsIndex_r4/Logical  logical_function=OR  inputs=9  en=off  latency=0  precision=Full  arith_type=Unsigned  n_bits=16  bin_pt=0  align_bp=on  dbl_ovrd=off  block_type=logical
  Logical8 : xbsIndex_r4/Logical  logical_function=AND  inputs=9  en=off  latency=0  precision=Full  arith_type=Unsigned  n_bits=16  bin_pt=0  align_bp=on  dbl_ovrd=off  block_type=logical
  Logical9 : xbsIndex_r4/Logical  logical_function=OR  inputs=9  en=off  latency=0  precision=Full  arith_type=Unsigned  n_bits=16  bin_pt=0  align_bp=on  dbl_ovrd=off  block_type=logical
  S-R Latch : Subsystem
  bool2 : xbsIndex_r4/Convert  gui_display_data_type=Boolean  arith_type=Boolean  n_bits=16  bin_pt=14  float_type=Single  exp_bits=8  fraction_bits=24  quantization=Truncate  overflow=Wrap  en=off  latency=0  dbl_ovrd=off  pipeline=off  block_type=convert
  Out : Outport
  tag scope: OUT2=global
  wires:
  [OUT2_AND_USE_IN0] -> Expression2/1, Logical12/1
  [OUT2_AND_USE_IN1] -> Expression1/1, Logical12/2
  [OUT2_AND_USE_IN2] -> Expression3/1, Logical12/3
  [OUT2_AND_USE_IN3] -> Expression4/1, Logical12/4
  [OUT2_AND_USE_IN4] -> Expression6/1, Logical12/5
  [OUT2_AND_USE_IN5] -> Expression5/1, Logical12/6
  [OUT2_AND_USE_IN6] -> Expression7/1, Logical12/7
  [OUT2_AND_USE_IN7] -> Expression8/1, Logical12/8
  In0/1 -> Logical/2, Expression2/2
  In1/1 -> Expression1/2, Logical1/2
  In2/1 -> Expression3/2, Logical2/2
  In3/1 -> Expression4/2, Logical3/2
  In4/1 -> Expression6/2, Logical4/2
  In5/1 -> Expression5/2, Logical5/2
  In6/1 -> Expression7/2, Logical6/2
  In7/1 -> Expression8/2, Logical7/2
  [OUT2_OR_USE_IN0] -> Logical/1
  [OUT2_OR_USE_IN1] -> Logical1/1
  Expression2/1 -> Logical8/1
  Expression1/1 -> Logical8/2
  Expression3/1 -> Logical8/3
  Expression4/1 -> Logical8/4
  Expression6/1 -> Logical8/5
  Expression5/1 -> Logical8/6
  Expression7/1 -> Logical8/7
  Expression8/1 -> Logical8/8
  Logical/1 -> Logical9/1
  Logical1/1 -> Logical9/2
  Logical2/1 -> Logical9/3
  Logical3/1 -> Logical9/4
  Logical4/1 -> Logical9/5
  Logical5/1 -> Logical9/6
  Logical6/1 -> Logical9/7
  Logical7/1 -> Logical9/8
  Logical9/1 -> Logical10/2
  Logical10/1 -> S-R Latch/1(S), Logical11/1
  [OUT2_RESET] -> S-R Latch/2(R)
  S-R Latch/1(Q) -> [OUT2], bool2/1
  Logical11/1 -> Out/1
  bool2/1 -> Logical11/2
  Logical12/1 -> Logical15/2
  Logical15/1 -> Logical10/1
  [OUT2_AND_USE_IN8] -> Expression9/1, Logical12/9
  In8/1 -> Expression9/2, Logical14/2
  Logical8/1 -> Logical15/1
  Expression9/1 -> Logical8/9
  [OUT2_OR_USE_IN2] -> Logical2/1
  [OUT2_OR_USE_IN3] -> Logical3/1
  [OUT2_OR_USE_IN4] -> Logical4/1
  [OUT2_OR_USE_IN5] -> Logical5/1
  [OUT2_OR_USE_IN6] -> Logical6/1
  [OUT2_OR_USE_IN7] -> Logical7/1
  [OUT2_OR_USE_IN8] -> Logical14/1
  Logical14/1 -> Logical9/9

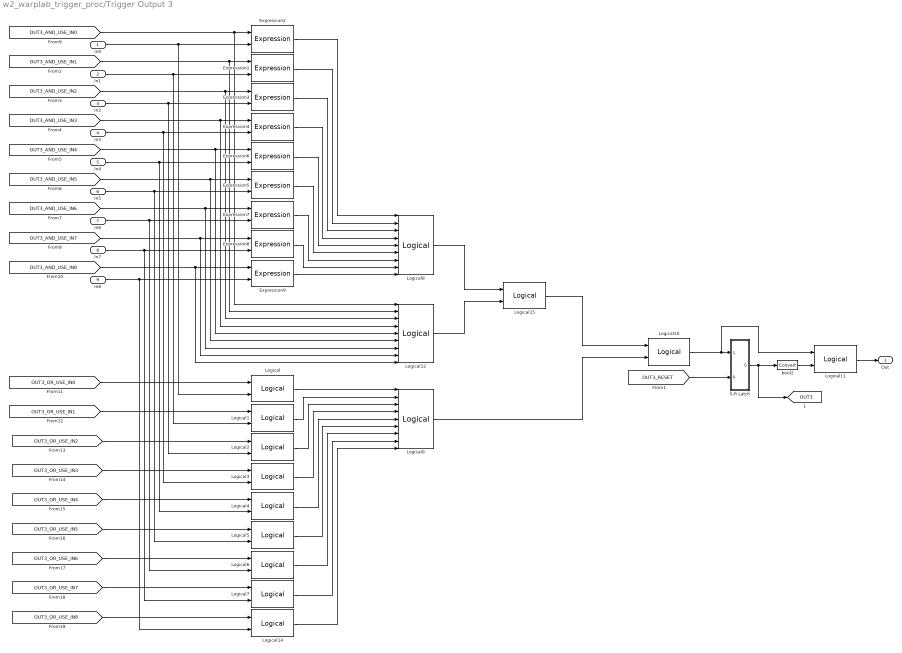
== system w2_warplab_trigger_proc/Trigger Output 3 ==
  In0 : Inport
  In1 : Inport  Port=2
  In2 : Inport  Port=3
  In3 : Inport  Port=4
  In4 : Inport  Port=5
  In5 : Inport  Port=6
  In6 : Inport  Port=7
  In7 : Inport  Port=8
  In8 : Inport  Port=9
  Expression{1..9} (9 alike) : xbsIndex_r4/Expression  expression=~a | (a & b)  align_bp=on  en=off  latency=0  precision=Full  arith_type=Unsigned  n_bits=16  bin_pt=0  dbl_ovrd=off  block_type=expr
  Logical{,1..7,14..15} (10 alike) : xbsIndex_r4/Logical  logical_function=AND  inputs=2  en=off  latency=0  precision=Full  arith_type=Unsigned  n_bits=16  bin_pt=0  align_bp=on  dbl_ovrd=off  block_type=logical
  Logical10 : xbsIndex_r4/Logical  logical_function=OR  inputs=2  en=off  latency=0  precision=Full  arith_type=Unsigned  n_bits=16  bin_pt=0  align_bp=on  dbl_ovrd=off  block_type=logical
  Logical11 : xbsIndex_r4/Logical  logical_function=OR  inputs=2  en=off  latency=0  precision=Full  arith_type=Unsigned  n_bits=16  bin_pt=0  align_bp=on  dbl_ovrd=off  block_type=logical
  Logical12 : xbsIndex_r4/Logical  logical_function=OR  inputs=9  en=off  latency=0  precision=Full  arith_type=Unsigned  n_bits=16  bin_pt=0  align_bp=on  dbl_ovrd=off  block_type=logical
  Logical8 : xbsIndex_r4/Logical  logical_function=AND  inputs=9  en=off  latency=0  precision=Full  arith_type=Unsigned  n_bits=16  bin_pt=0  align_bp=on  dbl_ovrd=off  block_type=logical
  Logical9 : xbsIndex_r4/Logical  logical_function=OR  inputs=9  en=off  latency=0  precision=Full  arith_type=Unsigned  n_bits=16  bin_pt=0  align_bp=on  dbl_ovrd=off  block_type=logical
  S-R Latch : Subsystem
  bool2 : xbsIndex_r4/Convert  gui_display_data_type=Boolean  arith_type=Boolean  n_bits=16  bin_pt=14  float_type=Single  exp_bits=8  fraction_bits=24  quantization=Truncate  overflow=Wrap  en=off  latency=0  dbl_ovrd=off  pipeline=off  block_type=convert
  Out : Outport
  tag scope: OUT3=global
  wires:
  [OUT3_AND_USE_IN0] -> Expression2/1, Logical12/1
  [OUT3_AND_USE_IN1] -> Expression1/1, Logical12/2
  [OUT3_AND_USE_IN2] -> Expression3/1, Logical12/3
  [OUT3_AND_USE_IN3] -> Expression4/1, Logical12/4
  [OUT3_AND_USE_IN4] -> Expression6/1, Logical12/5
  [OUT3_AND_USE_IN5] -> Expression5/1, Logical12/6
  [OUT3_AND_USE_IN6] -> Expression7/1, Logical12/7
  [OUT3_AND_USE_IN7] -> Expression8/1, Logical12/8
  In0/1 -> Logical/2, Expression2/2
  In1/1 -> Expression1/2, Logical1/2
  In2/1 -> Expression3/2, Logical2/2
  In3/1 -> Expression4/2, Logical3/2
  In4/1 -> Expression6/2, Logical4/2
  In5/1 -> Expression5/2, Logical5/2
  In6/1 -> Expression7/2, Logical6/2
  In7/1 -> Expression8/2, Logical7/2
  [OUT3_OR_USE_IN0] -> Logical/1
  [OUT3_OR_USE_IN1] -> Logical1/1
  Expression2/1 -> Logical8/1
  Expression1/1 -> Logical8/2
  Expression3/1 -> Logical8/3
  Expression4/1 -> Logical8/4
  Expression6/1 -> Logical8/5
  Expression5/1 -> Logical8/6
  Expression7/1 -> Logical8/7
  Expression8/1 -> Logical8/8
  Logical/1 -> Logical9/1
  Logical1/1 -> Logical9/2
  Logical2/1 -> Logical9/3
  Logical3/1 -> Logical9/4
  Logical4/1 -> Logical9/5
  Logical5/1 -> Logical9/6
  Logical6/1 -> Logical9/7
  Logical7/1 -> Logical9/8
  Logical9/1 -> Logical10/2
  Logical10/1 -> S-R Latch/1(S), Logical11/1
  [OUT3_RESET] -> S-R Latch/2(R)
  S-R Latch/1(Q) -> [OUT3], bool2/1
  Logical11/1 -> Out/1
  bool2/1 -> Logical11/2
  Logical12/1 -> Logical15/2
  Logical15/1 -> Logical10/1
  [OUT3_AND_USE_IN8] -> Expression9/1, Logical12/9
  In8/1 -> Expression9/2, Logical14/2
  Logical8/1 -> Logical15/1
  Expression9/1 -> Logical8/9
  [OUT3_OR_USE_IN2] -> Logical2/1
  [OUT3_OR_USE_IN3] -> Logical3/1
  [OUT3_OR_USE_IN4] -> Logical4/1
  [OUT3_OR_USE_IN5] -> Logical5/1
  [OUT3_OR_USE_IN6] -> Logical6/1
  [OUT3_OR_USE_IN7] -> Logical7/1
  [OUT3_OR_USE_IN8] -> Logical14/1
  Logical14/1 -> Logical9/9
